simulink model "GroupWork_ValerieLovesBuckConverter_Controller1"  (R2021b)
settings: Solver=FixedStepDiscrete  StartTime=0.0  StopTime=0.25  RelTol=1e-3
PreLoadFcn:
  | %
  | Fc=3780;                          % PWM Carrier frequency (Hz)
  | Ts_Power=1/Fc/200;         % Simscape Power Systems sample time (s)
  | Ts_Control=20*Ts_Power;  % Inverter Control system sample time (s)
InitFcn:
  | %
  | Fc=3780;                          % PWM Carrier frequency (Hz)
  | Ts_Power=1/Fc/200;         % Simscape Power Systems sample time (s)
  | Ts_Control=20*Ts_Power;  % Inverter Control system sample time (s)
undefined symbols (not defined in the file): Ion, Lithium
libraries: spsSeriesRLCBranchLib x4, spsDiodeLib x3, visionstatistics x2, spsMosfetLib x2, spsPWMGeneratorDCDCLib x2, spsStairGeneratorLib x2, spsPVArrayLib x2, spsBatteryLib x1, spsCurrentMeasurementLib x1, spsVoltageMeasurementLib x1, spspowerguiLib x1
Description:
  | Copyright 2008-2019 The MathWorks, Inc.
settings Model: Creator=MathWorks  LastModifiedBy=SWIFT3
settings SolverCC: AlgebraicLoopSolver=TrustRegion
settings DataIOCC: SaveFormat=Structure  SignalLoggingSaveFormat=ModelDataLogs  SaveOutput=off  SignalLogging=off  DSMLogging=off  SaveTime=off  ReturnWorkspaceOutputs=off
settings OptimizationCC: ExpressionDepthLimit=2147483647  LifeSpan=inf
settings DebuggingCC: UnderspecifiedInitializationDetection=Classic  MergeDetectMultiDrivingBlocksExec=none  SolverPrmCheckMsg=warning  FcnCallInpInsideContextMsg=warning  AllowSymbolicDim=off  StateNameClashWarn=warning  SFUnexpectedBacktrackingDiag=warning  SFNoUnconditionalDefaultTransitionDiag=warning  SFExecutionAtInitializationDiag=none  SFMachineParentedDataDiag=warning  ArithmeticOperatorsInVariantConditions=warning
settings HardwareCC: ProdBitPerPointer=32  ProdBitPerSizeT=32  ProdBitPerPtrDiffT=32  ProdLargestAtomicFloat=None  ProdIntDivRoundTo=Undefined  ProdEndianess=Unspecified  ProdWordSize=32  ProdHWDeviceType=32-bit Generic
settings ModelReferenceCC: PropagateSignalLabelsOutOfModel=off
settings SFSimCC: SimUseLocalCustomCode=off  CustomCodeUndefinedFunction=UseInterfaceOnly
settings RTWCC: RTWUseLocalCustomCode=off
settings CodeAppCC: StateflowObjectComments=on
settings GRTTargetCC: TargetLangStandard=C89/C90 (ANSI)  CombineOutputUpdateFcns=off  GRTInterface=on
settings ConfigComp: CovMetricSettings=dw  CovSaveCumulativeToWorkspaceVar=on  CovSaveSingleToWorkspaceVar=on  CovExternalEMLEnable=off  CovSFcnEnable=off
settings SimscapeCC: SimscapeNormalizeSystem=off

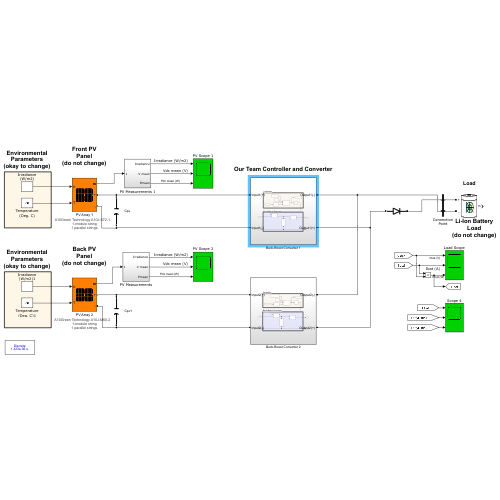
[thumbnail: Simulink's stored preview of the top-level diagram]
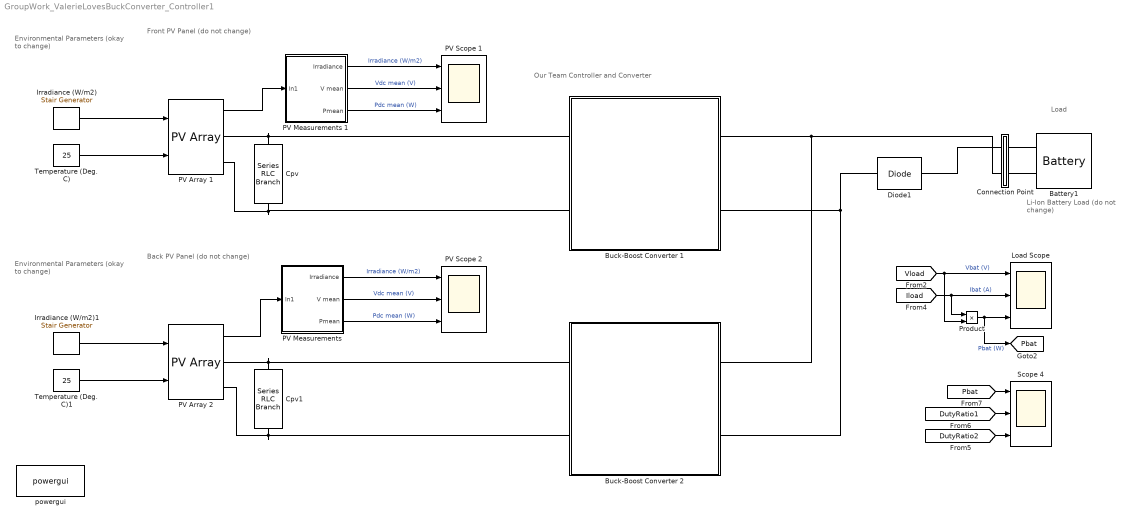
== system GroupWork_ValerieLovesBuckConverter_Controller1 ==
  note: Load
  note: Li-Ion Battery
      | Load
      | (do not change)
  note: Front PV
      | Panel
      | (do not change)
  note: Environmental
      | Parameters
      | (okay to change)
  note: Our Team Controller and Converter
  note: Environmental
      | Parameters
      | (okay to change)
  note: Back PV
      | Panel
      | (do not change)
  Battery1 : spsBatteryLib/Battery  BatType=Lithium-Ion  ShowTempParam=off  ThermalPreset=no  ShowAgeParam=off  NomV=100  NomQ=5  SOC=50  Batt_Tr=30  PresetModel=on  MaxQ=5  MinV=75  FullV=116.3987  Dis_rate=2.1739  R=0.2  Normal_OP=4.5217  expZone="[108.0386     0.2456522]"  current=[6.5 13 32.5]  Units=Time  Tci=20  NomT=20  T2=-30  MaxQ2=4.8  FullV2=7.1  Normal_OP2=5.655  expZone2="[6.58           1]"  Rca=0.6  ti=2000  Dp=0  Neq0=0  Tsim=1e6  Ta1=25  Qeol=5.4*0.9  Reol=0.013333*1.2  Char_age=[2.3478, 3]  Dis_age=[2.3478, 10]  N1=1500  N2=10500  N3=1000  N4=1400  Ta2=45  N5=950
  Buck-Boost Converter 1 : Subsystem
  Buck-Boost Converter 2 : Subsystem
  Connection Point : Subsystem
  Cpv : spsSeriesRLCBranchLib/Series RLC Branch  LConnTagsString=__new0  RConnTagsString=__new0  BranchType=C  Resistance=1  Inductance=1e-3  SetiL0=off  InitialCurrent=0  Capacitance=1e-5  Setx0=on  InitialVoltage=36  Measurements=None
  Cpv1 : spsSeriesRLCBranchLib/Series RLC Branch  LConnTagsString=__new0  RConnTagsString=__new0  BranchType=C  Resistance=1  Inductance=1e-3  SetiL0=off  InitialCurrent=0  Capacitance=1e-5  Setx0=on  InitialVoltage=36  Measurements=None
  Diode1 : spsDiodeLib/Diode  Ron=0.000000001  Lon=0  Vf=0  IC=0  UseSnubber=0  Rs=0  Cs=0  Measurements=off
  Irradiance (W/m2) : spsStairGeneratorLib/Stair Generator  t=0  e=1000  Ts=Ts_Power
  Irradiance (W/m2)1 : spsStairGeneratorLib/Stair Generator  t=0  e=1000  Ts=Ts_Power
  Load Scope : Scope  NumInputPorts=3
  PV Array 1 : spsPVArrayLib/PV Array  Npar=1  Nser=1  PlotType=array @ 1000 W/m2 & specified temperatures  S_vec="[ 1000  500  100 ]"  Temp_C_vec=[ 45 25 100 ]  ModuleName=A10Green Technology A10J-S72-175  PlotWhenSelected=off  Pm=175.0914  Ncell=72  Voc=43.99  Isc=5.17  Vm=36.63  Im=4.78  beta_Voc_pc=-0.3616  alpha_Isc_pc=0.041509  beta_Voc=-0.15907  alpha_Isc=0.002146  IL=5.178  I0=1.7842e-10  nI=0.98852  Rsh=249.6758  Rs=0.38412  RobustModel=off  RobustCellTemperature=313.3991  BAL=on  Tc=1e-6  Tfilter=5e-5
      settings: AttributesFormatString=|
      | %<ModuleName>
      | %<Nser>-module string
      | %<Npar> parallel strings
  PV Array 2 : spsPVArrayLib/PV Array  Npar=1  Nser=1  PlotType=array @ 1000 W/m2 & specified temperatures  S_vec="[ 1000  500  100 ]"  Temp_C_vec=[ 45 25 100 ]  ModuleName=A10Green Technology A10J-M60-240  PlotWhenSelected=off  Pm=240.5376  Ncell=60  Voc=36.84  Isc=8.32  Vm=30.72  Im=7.83  beta_Voc_pc=-0.359  alpha_Isc_pc=0.096995  beta_Voc=-0.13226  alpha_Isc=0.00807  IL=8.3299  I0=2.8736e-10  nI=0.99259  Rsh=330.6558  Rs=0.19366  RobustModel=off  RobustCellTemperature=313.3991  BAL=on  Tc=1e-6  Tfilter=5e-5
      settings: AttributesFormatString=|
      | %<ModuleName>
      | %<Nser>-module string
      | %<Npar> parallel strings
  PV Measurements : Subsystem
  PV Measurements 1 : Subsystem
  PV Scope 1 : Scope  NumInputPorts=3
  PV Scope 2 : Scope  NumInputPorts=3
  Product : Product
  Scope 4 : Scope  NumInputPorts=3
  Temperature (Deg. C) : Constant  Value=25
  Temperature (Deg. C)1 : Constant  Value=25
  powergui : spspowerguiLib/powergui  Priority=1  SimulationMode=Discrete  SampleTime=Ts_Power  frequency=60  Iterations=50  frequencyindice=0  Pbase=100e6  ErrMax=1e-4  UnitsV=kV  UnitsW=MW  buscounter=0  FunctionMessages=off  echomessages=off  EnableUseOfTLC=off  CurrentSourceSwitches=off  DisableSnubberDevices=off  DisableRonSwitches=off  DisableVfSwitches=off  DisplayEquations=off  AutomaticDiscreteSolvers=off  SolverType=Tustin/Backward Euler (TBE)  Interpol=off  ExternalGateDelay=off  methode=off  Ts=0  x0status=blocks  SPID=off  SwTol=0  HookPort=off  NonlinearTolerance=0  nMaxIteration=15  ContinueOnMaxIteration=off  RestoreLinks=warning  ResistiveCurrentMeasurement=off  Frange=[0:2:500]  Ylog=off  Xlog=on  ShowGrid=off  save=off  variable=ZData  structure=VIgrid  ZoomFFT=off  StartTime=0.55  cycles=1  DisplayStyle=1  fundamental=60  FreqAxis=on  MaxFrequency=10000  frequencyindicesteady=1  RmsSteady=1  display=off
  tag scope: Pbat=global
  wires:
  [Iload] -> Product/1, Load Scope/2  "Ibat (A)"
  Irradiance (W/m2)/1 -> PV Array 1/1
  Temperature (Deg. C)/1 -> PV Array 1/2
  PV Array 1/1 -> PV Measurements 1/1(In1)
  PV Measurements/2(V mean) -> PV Scope 2/2  "Vdc mean (V)"
  PV Measurements/1(Irradiance) -> PV Scope 2/1  "Irradiance (W/m2)"
  [Vload] -> Load Scope/1, Product/2  "Vbat (V)"
  Product/1 -> [Pbat], Load Scope/3  "Pbat (W)"
  PV Measurements/3(Pmean) -> PV Scope 2/3  "Pdc mean (W)"
  PV Array 2/1 -> PV Measurements/1(In1)
  Temperature (Deg. C)1/1 -> PV Array 2/2
  Irradiance (W/m2)1/1 -> PV Array 2/1
  PV Measurements 1/1(Irradiance) -> PV Scope 1/1  "Irradiance (W/m2)"
  PV Measurements 1/3(Pmean) -> PV Scope 1/3  "Pdc mean (W)"
  PV Measurements 1/2(V mean) -> PV Scope 1/2  "Vdc mean (V)"
  [DutyRatio2] -> Scope 4/3
  [DutyRatio1] -> Scope 4/2
  [Pbat] -> Scope 4/1
  connections:
  Connection Point/RConn1 -- Battery1/LConn1
  Connection Point/RConn2 -- Battery1/LConn2
  Cpv/LConn1 -- PV Array 1/RConn1 -- Buck-Boost Converter 1/LConn1
  Cpv/RConn1 -- Buck-Boost Converter 1/LConn2 -- PV Array 1/RConn2
  Cpv1/LConn1 -- Buck-Boost Converter 2/LConn1 -- PV Array 2/RConn1
  Buck-Boost Converter 2/LConn2 -- PV Array 2/RConn2 -- Cpv1/RConn1
  Buck-Boost Converter 2/RConn1 -- Connection Point/LConn2 -- Buck-Boost Converter 1/RConn1
  Buck-Boost Converter 1/RConn2 -- Diode1/LConn1 -- Buck-Boost Converter 2/RConn2
  Diode1/RConn1 -- Connection Point/LConn1

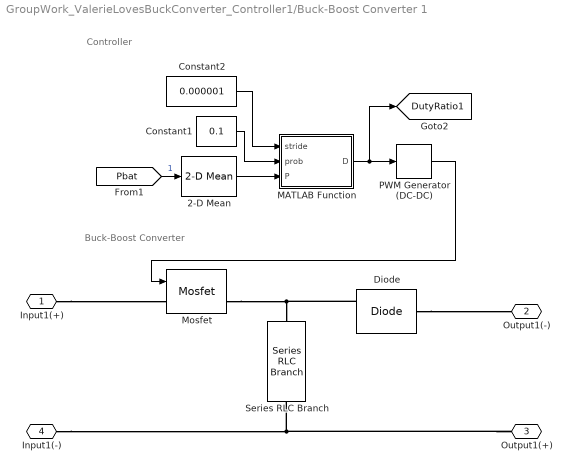
== system GroupWork_ValerieLovesBuckConverter_Controller1/Buck-Boost Converter 1 ==
  note: Controller
  note: Buck-Boost Converter
  2-D Mean : visionstatistics/2-D Mean  run=on  reset_popup=None  directionMode=Entire input  dimension=1  treatSBRowAsCol=on  outputLastDataTypeStr=Inherit: Same as accumulator  accumMode=Binary point scaling  accumWordLength=32  accumFracLength=0  accumLastDataTypeStr=fixdt([],32,0)  roiEnable=off  roiType=Rectangles  roiPortion=Entire ROI  roiOutput=Individual statistics for each ROI  roiFlag=off  roundingMode=Floor  overflowMode=off  accumDataTypeStr=fixdt([],32,0)  outputDataTypeStr=Inherit: Same as accumulator  outputMin=[]  outputMax=[]
      settings: SourceProductBaseCode=VP
  Constant1 : Constant  Value=0.1
  Constant2 : Constant  Value=0.000001
  Diode : spsDiodeLib/Diode  Ron=0.000000001  Lon=0  Vf=0.8  IC=0  UseSnubber=0  Rs=500  Cs=250e-9  Measurements=on
  MATLAB Function : MATLAB Function  TreatAsAtomicUnit=on
  Mosfet : spsMosfetLib/Mosfet  Ron=0.1  Lon=0  Rd=0.01  Vfd=0  IC=0  Rs=1e5  Cs=inf  Measurements=on
  PWM Generator (DC-DC) : spsPWMGeneratorDCDCLib/PWM Generator (DC-DC)  Fsw=50000  Ts=0
  Series RLC Branch : spsSeriesRLCBranchLib/Series RLC Branch  LConnTagsString=__new0  RConnTagsString=__new0  BranchType=L  Resistance=1  Inductance=1e-3  SetiL0=off  InitialCurrent=0  Capacitance=1e-6  Setx0=off  InitialVoltage=0  Measurements=None
  Input1(+) : PMIOPort  Side=Left
  Output1(-) : PMIOPort  Port=2  Side=Right
  Output1(+) : PMIOPort  Port=3  Side=Right
  Input1(-) : PMIOPort  Port=4  Side=Left
  tag scope: DutyRatio1=global
  wires:
  PWM Generator (DC-DC)/1 -> Mosfet/1
  MATLAB Function/1(D) -> [DutyRatio1], PWM Generator (DC-DC)/1
  [Pbat] -> 2-D Mean/1  "1"
  2-D Mean/1 -> MATLAB Function/3(P)
  Constant1/1 -> MATLAB Function/2(prob)
  Constant2/1 -> MATLAB Function/1(stride)
  connections:
  Diode/LConn1 -- Output1(-)/RConn1
  Mosfet/RConn1 -- Diode/RConn1 -- Series RLC Branch/LConn1
  Input1(+)/RConn1 -- Mosfet/LConn1
  Output1(+)/RConn1 -- Input1(-)/RConn1 -- Series RLC Branch/RConn1

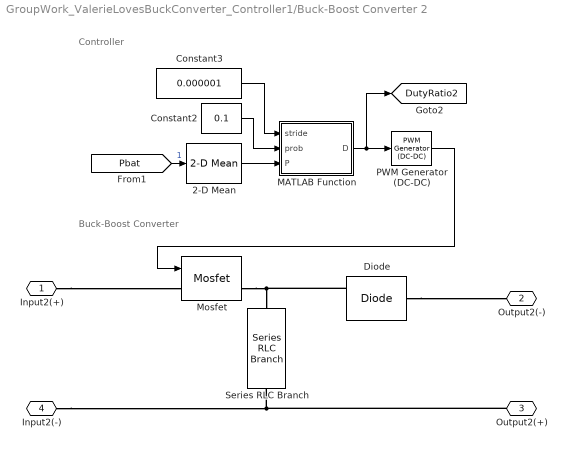
== system GroupWork_ValerieLovesBuckConverter_Controller1/Buck-Boost Converter 2 ==
  note: Controller
  note: Buck-Boost Converter
  2-D Mean : visionstatistics/2-D Mean  run=on  reset_popup=None  directionMode=Entire input  dimension=1  treatSBRowAsCol=on  outputLastDataTypeStr=Inherit: Same as accumulator  accumMode=Binary point scaling  accumWordLength=32  accumFracLength=0  accumLastDataTypeStr=fixdt([],32,0)  roiEnable=off  roiType=Rectangles  roiPortion=Entire ROI  roiOutput=Individual statistics for each ROI  roiFlag=off  roundingMode=Floor  overflowMode=off  accumDataTypeStr=fixdt([],32,0)  outputDataTypeStr=Inherit: Same as accumulator  outputMin=[]  outputMax=[]
      settings: SourceProductBaseCode=VP
  Constant2 : Constant  Value=0.1
  Constant3 : Constant  Value=0.000001
  Diode : spsDiodeLib/Diode  Ron=0.00000001  Lon=0  Vf=0.8  IC=0  UseSnubber=0  Rs=500  Cs=250e-9  Measurements=on
  MATLAB Function : MATLAB Function  TreatAsAtomicUnit=on
  Mosfet : spsMosfetLib/Mosfet  Ron=0.1  Lon=0  Rd=0.01  Vfd=0  IC=0  Rs=1e5  Cs=inf  Measurements=on
  PWM Generator (DC-DC) : spsPWMGeneratorDCDCLib/PWM Generator (DC-DC)  Fsw=50000  Ts=0
  Series RLC Branch : spsSeriesRLCBranchLib/Series RLC Branch  LConnTagsString=__new0  RConnTagsString=__new0  BranchType=L  Resistance=1  Inductance=1e-3  SetiL0=off  InitialCurrent=0  Capacitance=1e-6  Setx0=off  InitialVoltage=0  Measurements=None
  Input2(+) : PMIOPort  Side=Left
  Output2(-) : PMIOPort  Port=2  Side=Right
  Output2(+) : PMIOPort  Port=3  Side=Right
  Input2(-) : PMIOPort  Port=4  Side=Left
  tag scope: DutyRatio2=global
  wires:
  PWM Generator (DC-DC)/1 -> Mosfet/1
  2-D Mean/1 -> MATLAB Function/3(P)
  [Pbat] -> 2-D Mean/1  "1"
  MATLAB Function/1(D) -> [DutyRatio2], PWM Generator (DC-DC)/1
  Constant2/1 -> MATLAB Function/2(prob)
  Constant3/1 -> MATLAB Function/1(stride)
  connections:
  Diode/LConn1 -- Output2(-)/RConn1
  Mosfet/RConn1 -- Series RLC Branch/LConn1 -- Diode/RConn1
  Input2(+)/RConn1 -- Mosfet/LConn1
  Output2(+)/RConn1 -- Input2(-)/RConn1 -- Series RLC Branch/RConn1

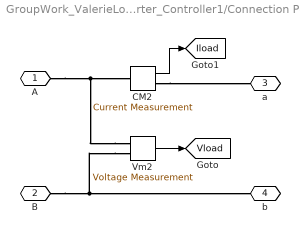
== system GroupWork_ValerieLovesBuckConverter_Controller1/Connection Point ==
  CM2 : spsCurrentMeasurementLib/Current Measurement  PhasorSimulation=off  OutputType=Complex  PSBequivalent=0
  Vm2 : spsVoltageMeasurementLib/Voltage Measurement  PhasorSimulation=off  OutputType=Complex  PSBequivalent=0
  A : PMIOPort  Side=Left
  B : PMIOPort  Port=2  Side=Left
  a : PMIOPort  Port=3  Side=Right
  b : PMIOPort  Port=4  Side=Right
  tag scope: Iload=global, Vload=global
  wires:
  Vm2/1 -> [Vload]
  CM2/1 -> [Iload]
  connections:
  Vm2/LConn2 -- b/RConn1 -- B/RConn1
  Vm2/LConn1 -- A/RConn1 -- CM2/LConn1
  CM2/RConn1 -- a/RConn1

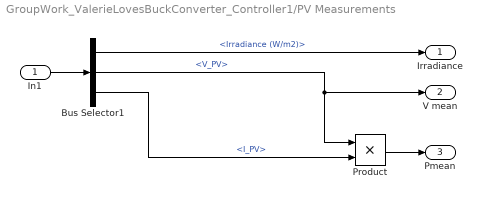
== system GroupWork_ValerieLovesBuckConverter_Controller1/PV Measurements ==
  In1 : Inport
  Bus Selector1 : BusSelector  OutputSignals=Irradiance (W/m2),V_PV,I_PV
  Product : Product
  Irradiance : Outport  VectorParamsAs1DForOutWhenUnconnected=off
  V mean : Outport  Port=2  VectorParamsAs1DForOutWhenUnconnected=off
  Pmean : Outport  Port=3  VectorParamsAs1DForOutWhenUnconnected=off
  wires:
  In1/1 -> Bus Selector1/1
  Bus Selector1/2 -> Product/1, V mean/1  "<V_PV>"
  Bus Selector1/3 -> Product/2  "<I_PV>"
  Bus Selector1/1 -> Irradiance/1  "<Irradiance (W/m2)>"
  Product/1 -> Pmean/1

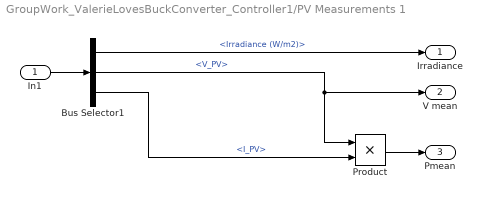
== system GroupWork_ValerieLovesBuckConverter_Controller1/PV Measurements 1 ==
  In1 : Inport
  Bus Selector1 : BusSelector  OutputSignals=Irradiance (W/m2),V_PV,I_PV
  Product : Product
  Irradiance : Outport  VectorParamsAs1DForOutWhenUnconnected=off
  V mean : Outport  Port=2  VectorParamsAs1DForOutWhenUnconnected=off
  Pmean : Outport  Port=3  VectorParamsAs1DForOutWhenUnconnected=off
  wires:
  In1/1 -> Bus Selector1/1
  Bus Selector1/2 -> Product/1, V mean/1  "<V_PV>"
  Bus Selector1/3 -> Product/2  "<I_PV>"
  Bus Selector1/1 -> Irradiance/1  "<Irradiance (W/m2)>"
  Product/1 -> Pmean/1

== matlab function GroupWork_ValerieLovesBuckConverter_Controller1/Buck-Boost Converter 2/MATLAB Function ==
  data: stride input; prob input; P input; D output
function D = fcn(stride, prob, P)
Dinit = 0.786;
deltaD = stride;
persistent Pold Dold LDD;
if isempty(Pold)
    Pold = 0;
    Dold = Dinit;
    LDD = 0;
else
end
D = Dold;
dP = P - Pold;
if dP ~= 0
    randnum = rand; 
    if dP < 0
        if (LDD > 0 & randnum > prob) | (LDD < 0 & randnum < prob)
            D = Dold - deltaD;
            LDD = -1;
        else
            D = Dold + deltaD;
            LDD = 1;
        end
    else
        if (LDD > 0 & randnum > prob) | (LDD < 0 & randnum < prob)
            D = Dold + deltaD;
            LDD = 1;
        else
            D = Dold - deltaD;
            LDD = -1;
        end
    end
end
if D >= 1 | D <= 0
    D = Dold;
else
end
Dold = D;
Pold = P;

== matlab function GroupWork_ValerieLovesBuckConverter_Controller1/Buck-Boost Converter 1/MATLAB Function ==
  data: stride input; prob input; P input; D output
function D = fcn(stride, prob, P)
Dinit = 0.749;
deltaD = stride;
persistent Pold Dold LDD;
if isempty(Pold)
    Pold = 0;
    Dold = Dinit;
    LDD = 0;
else
end
D = Dold;
dP = P - Pold;
if dP ~= 0
    randnum = rand; 
    if dP < 0
        if (LDD > 0 & randnum > prob) | (LDD < 0 & randnum < prob)
            D = Dold - deltaD;
            LDD = -1;
        else
            D = Dold + deltaD;
            LDD = 1;
        end
    else
        if (LDD > 0 & randnum > prob) | (LDD < 0 & randnum < prob)
            D = Dold + deltaD;
            LDD = 1;
        else
            D = Dold - deltaD;
            LDD = -1;
        end
    end
end
if D >= 1 | D <= 0
    D = Dold;
else
end
Dold = D;
Pold = P;
